simulink model "PickAndPlace_Simulation_QLabs"  (R2024a)
settings: Solver=FixedStepDiscrete  StartTime=0.0  StopTime=inf  FixedStep=0.005  RelTol=1e-3
InitFcn:
  | qarmRigidBodyTree = importrobot('Resources/qarm/urdf/QARM.urdf');
  | qarmRigidBodyTree.Bodies{1,3}.Joint.PositionLimits(1) = -pi/4;
  | show(qarmRigidBodyTree);
undefined symbols (not defined in the file): EFFECTOR, END, HIL, Levenberg, Marquardt, qc_get_step_size, Video3D
libraries: quarc_library x8, robotmaniplib x2, dspnetwork x1
settings Model: Creator=MLevis  LastModifiedBy=是旺旺哦~
settings DebuggingCC: UnconnectedInputMsg=warning  UnconnectedOutputMsg=warning  UnconnectedLineMsg=warning
settings ModelReferenceCC: EnableRefExpFcnMdlSchedulingChecks=on
settings RTWCC: GPUComputeCapability=3.5  DLArmComputeVersion=19.05

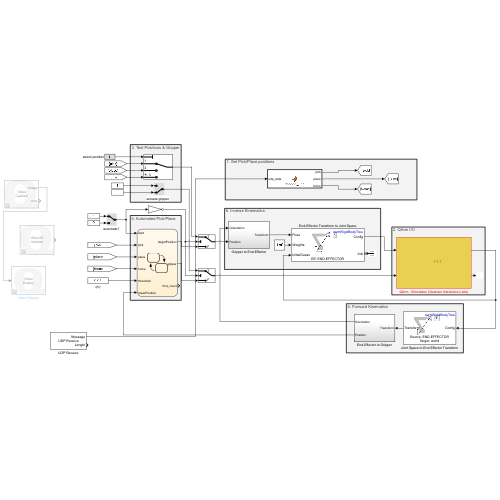
[thumbnail: Simulink's stored preview of the top-level diagram]
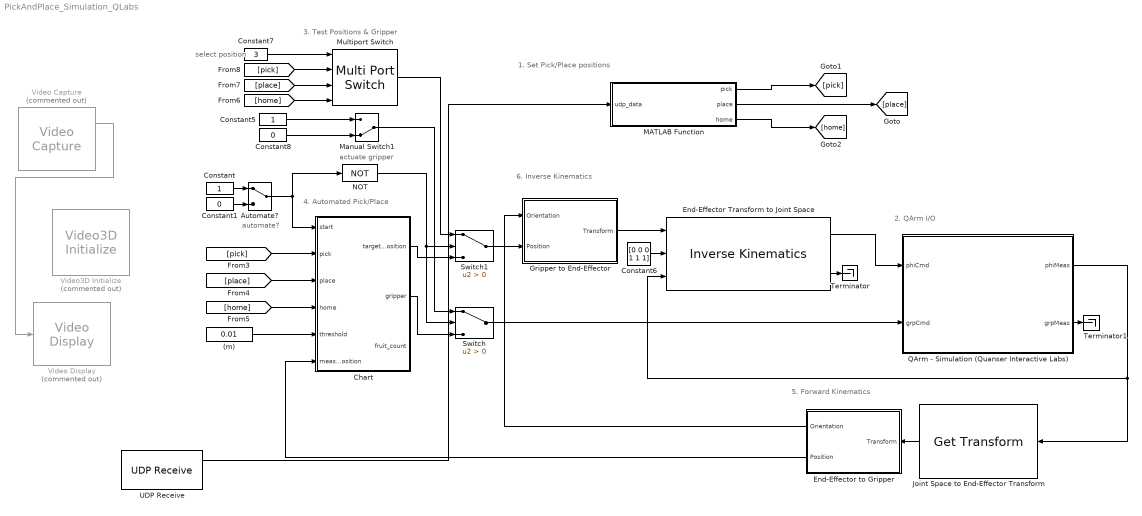
== system PickAndPlace_Simulation_QLabs ==
  note: 6. Inverse Kinematics
  note: 1. Set Pick/Place positions
  note: 4. Automated Pick/Place
  note: 2. QArm I/O
  note: 3. Test Positions & Gripper
  note: select position
  note: actuate gripper
  note: 5. Forward Kinematics
  note: automate?
  (m) : Constant  Value=0.01
  Automate? : ManualSwitch
  Chart : Stateflow chart  TreatAsAtomicUnit=on
  Constant : Constant
  Constant1 : Constant  Value=0
  Constant5 : Constant
  Constant6 : Constant  Value=[0 0 0 1 1 1]
  Constant7 : Constant  Value=3
  Constant8 : Constant  Value=0
  End-Effector Transform to Joint Space : robotmaniplib/Inverse Kinematics  RigidBodyTree=qarmRigidBodyTree  EndEffector=END-EFFECTOR  ShowInfo=on  SolverName=Levenberg-Marquardt  EnforceJointLimits=on  MaxIterations=2  MaxTime=qc_get_step_size  GradientTolerance=1e-4  SolutionTolerance=1e-3  StepTolerance=1e-3  ErrorChangeTolerance=1e-6  UseErrorDamping=on  DampingBias=0.0025  SimulateUsing=Code generation
  End-Effector to Gripper : Subsystem
  Gripper to End-Effector : Subsystem
  Joint Space to End-Effector Transform : robotmaniplib/Get Transform  RigidBodyTree=qarmRigidBodyTree  SourceBody=END-EFFECTOR  TargetBody=world  SimulateUsing=Interpreted execution
  MATLAB Function : MATLAB Function  TreatAsAtomicUnit=on
  Manual Switch1 : ManualSwitch  CurrentSetting=0
  Multiport Switch : MultiPortSwitch  SaturateOnIntegerOverflow=off  InputSameDT=off
  NOT : Logic  Operator=NOT  IconShape=distinctive  AllPortsSameDT=off  OutDataTypeStr=boolean
  QArm - Simulation (Quanser Interactive Labs) : Subsystem
      mask Display:
      | image('Resources/QArm.png')
      | port_label('input', 1, 'phiCmd');
      | port_label('input', 2, 'grpCmd');
      | port_label('output', 1, 'phiMeas');
      | port_label('output', 2, 'grpMeas');
  Switch : Switch  Criteria=u2 > Threshold  SaturateOnIntegerOverflow=off  InputSameDT=off
  Switch1 : Switch  Criteria=u2 > Threshold  SaturateOnIntegerOverflow=off  InputSameDT=off
  Terminator : Terminator
  Terminator1 : Terminator
  UDP Receive : dspnetwork/UDP Receive  localURL='0.0.0.0'  localPort=5000  remoteURL='0.0.0.0'  remotePort=-1  recvBufferSize=1024  dims=4  signalDatatype=double  isComplex=off  isVarSize=off  showBlockingTime=off  blockingTime=0  sampletime=0.02  blockPlatform=[]
      settings: LibrarySourceBlock=dspsrcs4/UDP Receive
  Video Capture : quarc_library/Multimedia/Video Capture  Commented=on  source=device  device=0  filename=sample_movie.mov  value=[0 0; 0 0]  resolution=640 x 480  width=640  height=480  output_format=MATLAB RGB (HxWx3)  data_type=uint8  sample_time=qc_get_step_size * ceil(0.033 / qc_get_step_size)  brightness_override=Do not override  brightness=50.0  contrast_override=Do not override  contrast=50.0  hue_override=Do not override  hue=50.0  saturation_override=Do not override  saturation=50.0  sharpness_override=Do not override  sharpness=50.0  gamma_override=Do not override  gamma=50.0  coloreffect_override=Do not override  coloreffect=None  whitebalance_override=Do not override  whitebalance=50.0  backlightcompensation_override=Do not override  backlightcompensation=0.0  gain_override=Do not override  gain=50.0  pan_override=Do not override  pan=50.0  tilt_override=Do not override  tilt=50.0  roll_override=Do not override  roll=50.0  zoom_override=Do not override  zoom=0.0  exposure_override=Do not override  exposure=50.0  iris_override=Do not override  iris=50.0  mirror_override=Do not override  mirror=None  focus_override=Do not override  focus=0.0
      settings: SourceProductName=QUARC Targets
  Video Display : quarc_library/Multimedia/Video Display  Tag=PickAndPlace_Simulation_QLabs/Video Display  Commented=on  sample_time=-1  use_hardware=on
  Video3D Initialize : quarc_library/Multimedia/Video3D Initialize  Commented=on  object_name=Video3D-1  source=Device  identifier=0  file=video3d://localhost:18001  sample_time=qc_get_step_size  active=on
  wires:
  End-Effector to Gripper/1(Orientation) -> Gripper to End-Effector/1(Orientation)
  [place] -> Multiport Switch/3
  Manual Switch1/1 -> Switch/1
  NOT/1 -> Switch1/2, Switch/2
  [home] -> Chart/4(home)
  QArm - Simulation (Quanser Interactive Labs)/1(phiMeas) -> End-Effector Transform to Joint Space/3, Joint Space to End-Effector Transform/1
  End-Effector Transform to Joint Space/2 -> Terminator/1
  Switch/1 -> QArm - Simulation (Quanser Interactive Labs)/2(grpCmd)
  [place] -> Chart/3(place)
  (m)/1 -> Chart/5(threshold)
  [pick] -> Chart/2(pick)
  Constant/1 -> Automate?/1
  Joint Space to End-Effector Transform/1 -> End-Effector to Gripper/1(Transform)
  QArm - Simulation (Quanser Interactive Labs)/2(grpMeas) -> Terminator1/1
  End-Effector to Gripper/2(Position) -> Chart/6(measPosition)
  End-Effector Transform to Joint Space/1 -> QArm - Simulation (Quanser Interactive Labs)/1(phiCmd)
  Constant8/1 -> Manual Switch1/2
  Automate?/1 -> NOT/1, Chart/1(start)
  Switch1/1 -> Gripper to End-Effector/2(Position)
  Constant6/1 -> End-Effector Transform to Joint Space/2
  Constant7/1 -> Multiport Switch/1
  Multiport Switch/1 -> Switch1/1
  Chart/1(targetPosition) -> Switch1/3
  Constant5/1 -> Manual Switch1/1
  Chart/2(gripper) -> Switch/3
  [pick] -> Multiport Switch/2
  [home] -> Multiport Switch/4
  Gripper to End-Effector/1(Transform) -> End-Effector Transform to Joint Space/1
  Constant1/1 -> Automate?/2
  MATLAB Function/1(pick) -> [pick]
  MATLAB Function/2(place) -> [place]
  MATLAB Function/3(home) -> [home]
  UDP Receive/1 -> MATLAB Function/1(udp_data)
  Video Capture/1 -> Video Display/1

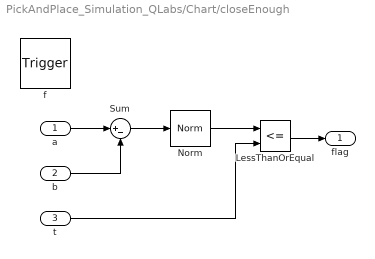
== system PickAndPlace_Simulation_QLabs/Chart/closeEnough ==
  a : Inport  OutDataTypeStr=double  PortDimensions=[3,1]
  b : Inport  Port=2  OutDataTypeStr=double  PortDimensions=[3,1]
  t : Inport  Port=3  OutDataTypeStr=double  PortDimensions=[1]
  f : TriggerPort  TriggerType=function-call  VariantControl=(inherit)
      settings: CopyFcn=Stateflow.SLINSF.SimulinkMan.removeBlockPreDeleteFcn  PreDeleteFcn=Stateflow.SLINSF.SimulinkMan.unsafePredeleteFcn
  LessThanOrEqual : RelationalOperator  Operator=<=  OutDataTypeStr=boolean  RndMeth=Simplest  InputSameDT=off
  Norm : quarc_library/Math Operations/Vectors/Norm
      settings: SourceProductName=QUARC Targets
  Sum : Sum  Inputs=|+-
  flag : Outport  VectorParamsAs1DForOutWhenUnconnected=off
  wires:
  a/1 -> Sum/1
  b/1 -> Sum/2
  Sum/1 -> Norm/1
  Norm/1 -> LessThanOrEqual/1
  t/1 -> LessThanOrEqual/2
  LessThanOrEqual/1 -> flag/1

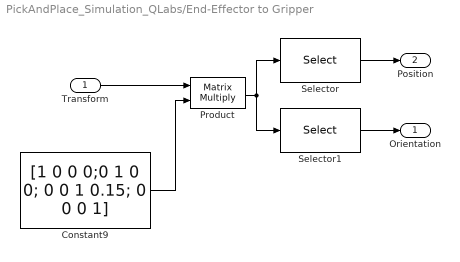
== system PickAndPlace_Simulation_QLabs/End-Effector to Gripper ==
  Transform : Inport
  Constant9 : Constant  Value=[1 0 0 0;0 1 0 0; 0 0 1 0.15; 0 0 0 1]  VectorParams1D=off
  Product : Product  Multiplication=Matrix(*)
  Selector : Selector  NumberOfDimensions=2  InputPortWidth=3  IndexOptions=Index vector (dialog),Index vector (dialog)  Indices=[1:3],4  OutputSizes=1,1
  Selector1 : Selector  NumberOfDimensions=2  InputPortWidth=3  IndexOptions=Index vector (dialog),Index vector (dialog)  Indices=[1:3],[1:3]  OutputSizes=1,1
  Orientation : Outport
  Position : Outport  Port=2
  wires:
  Transform/1 -> Product/1
  Product/1 -> Selector/1, Selector1/1
  Selector/1 -> Position/1
  Constant9/1 -> Product/2
  Selector1/1 -> Orientation/1

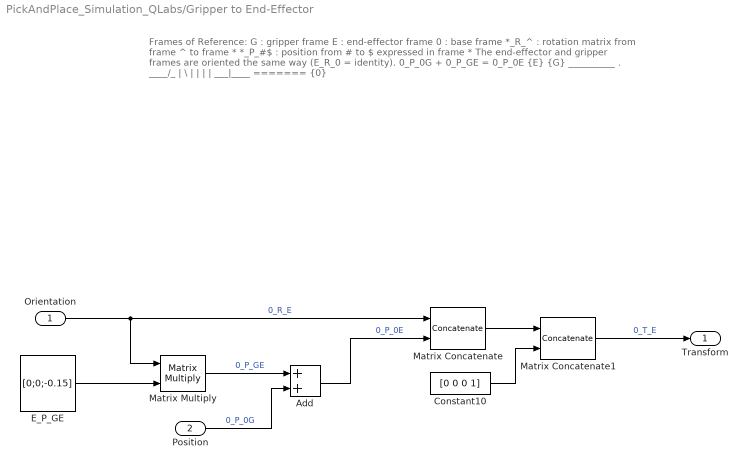
== system PickAndPlace_Simulation_QLabs/Gripper to End-Effector ==
  note: Frames of Reference:
      |
      | G : gripper frame
      | E : end-effector frame
      | 0 : base frame
      | *_R_^ : rotation matrix from frame ^ to frame *
      | *_P_#$ : position from # to $ expressed in frame *
      |
      | The end-effector and gripper frames are oriented the same way (E_R_0 = identity).
      | 0_P_0G + 0_P_GE = 0_P_0E
      |
      | {E} {G}
      | __________ . ____/_
      | | \
      | |
      | |
      | |
      | |
      | ___|____
      | =======
      | {0}
  Orientation : Inport
  Position : Inport  Port=2
  Add : Sum
  Constant10 : Constant  Value=[0 0 0 1]  VectorParams1D=off
  E_P_GE : Constant  Value=[0;0;-0.15]  VectorParams1D=off
  Matrix Concatenate : Concatenate  Mode=Multidimensional array  ConcatenateDimension=2
  Matrix Concatenate1 : Concatenate  Mode=Multidimensional array
  Matrix Multiply : Product  Multiplication=Matrix(*)
  Transform : Outport
  wires:
  Matrix Concatenate/1 -> Matrix Concatenate1/1
  Orientation/1 -> Matrix Concatenate/1, Matrix Multiply/1  "0_R_E"
  Constant10/1 -> Matrix Concatenate1/2
  Matrix Concatenate1/1 -> Transform/1  "0_T_E"
  Matrix Multiply/1 -> Add/1  "0_P_GE"
  Position/1 -> Add/2  "0_P_0G"
  E_P_GE/1 -> Matrix Multiply/2
  Add/1 -> Matrix Concatenate/2  "0_P_0E"

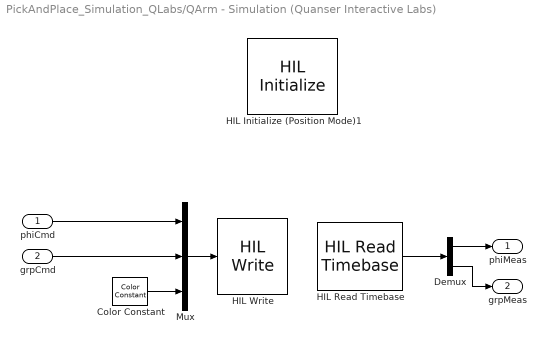
== system PickAndPlace_Simulation_QLabs/QArm - Simulation (Quanser Interactive Labs) ==
  phiCmd : Inport
  grpCmd : Inport  Port=2
  Color Constant : quarc_library/Sources/Signals/Color Constant  color=[0 1 0]
      settings: SourceProductName=QUARC Targets
  Demux : Demux  Outputs=[4 1]
  HIL Initialize (Position Mode)1 : quarc_library/Data Acquisition/Generic/Configuration/HIL Initialize  object_name=HIL-1  board_type=qarm_usb  board_number=0@tcpip://localhost:18900?nagle='off'  board_options=j0_mode=0;j1_mode=0;j2_mode=0;j3_mode=0;gripper_mode=0;  exclusive=off  active=on  hardware_clocks=[0]  clock_modes=[]  initial_clock_frequencies=[]  set_clock_params_at_start=off  set_clock_params_at_switch_in=off  set_clock_frequencies_at_start=off  set_clock_frequencies_at_switch_in=off  analog_input_channels=[5:9]  analog_input_configurations=[]  analog_input_maximums=[]  analog_input_minimums=[]  set_analog_input_params_at_start=off  set_analog_input_params_at_switch_in=off  analog_output_channels=[]  analog_output_maximums=inf  analog_output_minimums=-inf  initial_analog_outputs=[0]  final_analog_outputs=[0]  watchdog_analog_outputs=[]  set_analog_output_params_at_start=off  set_analog_output_params_at_switch_in=off  set_analog_outputs_at_start=off  set_analog_outputs_at_switch_in=off  set_analog_outputs_at_terminate=off  set_analog_outputs_at_switch_out=off  set_analog_outputs_on_watchdog=off  digital_input_channels=[]  digital_output_channels=[]  digital_output_configuration=[]  initial_digital_outputs=[0]  final_digital_outputs=[0]  watchdog_digital_outputs=[0]  set_digital_output_params_at_start=off  set_digital_output_params_at_switch_in=off  set_digital_outputs_at_start=off  set_digital_outputs_at_switch_in=off  set_digital_outputs_at_terminate=off  set_digital_outputs_at_switch_out=off  set_digital_outputs_on_watchdog=off  encoder_channels=[]  quadrature=[]  encoder_filter_frequency=[]  initial_encoder_counts=[]  set_encoder_params_at_start=off  set_encoder_params_at_switch_in=off  set_encoder_counts_at_start=off  set_encoder_counts_at_switch_in=off  pwm_channels=[]  pwm_modes=[]  pwm_frequency=[]  pwm_configuration=[]  pwm_alignment=[]  pwm_polarity=[]  pwm_leading_deadband=[]  pwm_trailing_deadband=[]  initial_pwm_outputs=[]  final_pwm_outputs=[]  watchdog_pwm_outputs=[]  set_pwm_params_at_start=off  set_pwm_params_at_switch_in=off  set_pwm_outputs_at_start=off  set_pwm_outputs_at_switch_in=off  set_pwm_outputs_at_terminate=off  set_pwm_outputs_at_switch_out=off  set_pwm_outputs_on_watchdog=off  other_output_channels=[1000:1004 11000:11003 11005:11007]  initial_other_outputs=[zeros(1,9), ones(1,3)]  final_other_outputs=[zeros(1,9), ones(1,3)]  watchdog_other_outputs=zeros(1,12)  set_other_outputs_at_start=off  set_other_outputs_at_switch_in=off  set_other_outputs_at_terminate=on  set_other_outputs_at_switch_out=off  set_other_outputs_on_watchdog=off
      settings: AttributesFormatString=%<object_name> (%<board_type>-%<board_number>)
  HIL Read Timebase : quarc_library/Data Acquisition/Generic/Timebases/HIL Read Timebase  object_name=HIL-1  clock=0  analog_channels=[]  encoder_channels=[]  digital_channels=[]  other_channels=[1000:1004]  active=on  vector_output=on  data_type_mode=Inherit via back propagation  encoder_data_type=double  digital_data_type=boolean  overflow_mode=Synchronize (for simulated cards only)  samples_in_buffer=max(ceil(1/qc_get_step_size), 1)
  HIL Write : quarc_library/Data Acquisition/Generic/Immediate I//O/HIL Write  object_name=HIL-1  analog_channels=[]  pwm_channels=[]  digital_channels=[]  other_channels=[1000:1004 11005:11007]  sample_time=-1  active=on  vector_input=on
  Mux : Mux  Inputs=3
  phiMeas : Outport
  grpMeas : Outport  Port=2
  wires:
  Mux/1 -> HIL Write/1
  grpCmd/1 -> Mux/2
  Color Constant/1 -> Mux/3
  HIL Read Timebase/1 -> Demux/1
  phiCmd/1 -> Mux/1
  Demux/1 -> phiMeas/1
  Demux/2 -> grpMeas/1

== matlab function PickAndPlace_Simulation_QLabs/MATLAB Function ==
  data: udp_data input; pick output; place output; home output
function [pick, place, home] = decode_udp(udp_data)
    % 1. Set the safety standby point (always a 3x1 vertical column vector)
    home = [0.45; 0; 0.49];
    
    % 2. Parse the 4 pieces of data sent by Python via UDP
    %Expected format:  udp_data = [X, Y, Z, Fruit_ID]
    x = udp_data(1);
    y = udp_data(2);
    z = udp_data(3);
    fruit_id = udp_data(4);
    
    % Security Protection: If Python has not yet sent any data, UDP will default to outputting 0. At this point, it will remain in its current position and wait.
    if x == 0 && y == 0 && z == 0
        pick = home;
    else
        pick = [x; y; z];
    end

    % 3. Intelligent classification and allocation (Determine the basket based on the Fruit_ID sent by Python) 
    if fruit_id == 1
        %  1 represents strawberry, add to Strawberry Pack
        place = [-0.45; 0.45; 0.38]; 
    elseif fruit_id == 2
        % 2 represents banana and it is placed in Basket A
        place = [0.0; 0.45; 0.38]; 
    elseif fruit_id == 3
        % 3 represents tomato, and it is placed in Basket B
        place = [0.45; 0.45; 0.38]; 
    else
        place = home; 
    end
end

== stateflow chart PickAndPlace_Simulation_QLabs/Chart ==
  state Wait
    en:
    gripper=0;
    targetPosition=home;
    fruit_count = 1;
  state flag = closeEnough(a,b,t) [function]
  state GotoPick
    targetPosition=pick;
    flag = closeEnough(measPosition, targetPosition, threshold);
  state CloseGripper
    gripper=1;
  state Done
    en:
    targetPosition = home;
  state GotoHome
    targetPosition=home;
    flag = closeEnough(measPosition, targetPosition, threshold);
  state GotoPlace
    targetPosition=place;
    flag = closeEnough(measPosition, targetPosition, threshold);
  state OpenGripper
    en:
    gripper=0;
    fruit_count = fruit_count + 1;
  (default) -> Wait
  Wait -> GotoPick : [start && after(2,sec)]
  GotoPick -> CloseGripper : [after(2,sec) && flag]
  CloseGripper -> GotoHome : [after(2,sec)]
  GotoHome -> GotoPick [order 2] : [after(2,sec) && flag && fruit_count <= 14]
  GotoHome -> GotoPlace [order 1] : [gripper && after(2,sec) && flag]
  OpenGripper -> GotoHome : [after(2,sec)]
  GotoHome -> Done [order 3] : [[after(2,sec) && flag && fruit_count > 14]]
  GotoPlace -> OpenGripper : [after(3,sec) && flag]
  data: a function_input double size=[3,1]; b function_input double size=[3,1]; flag function_output; t function_input double size=[1]; start input; pick input size=[3,1]; targetPosition output size=[3,1]; gripper output size=[1]; place input double size=[3,1]; home input double size=[3,1]; threshold input; measPosition input double size=[3,1]; flag local; fruit_count output
